simulink model "Disc_Integ_Forward_Euler_method_inherited_Sample_Time"  (R2014a)
settings: Solver=ode3  StartTime=0.0  StopTime=10.0  RelTol=1e-3
undefined symbols (not defined in the file): DiscIntNeverNeededParam
settings Model: CovSFcnEnable=on  Creator=bourbouh  LastModifiedBy=hbourbou
settings DataIOCC: LimitDataPoints=off  SaveFormat=StructureWithTime
settings DebuggingCC: MergeDetectMultiDrivingBlocksExec=error  SolverPrmCheckMsg=none  FrameProcessingCompatibilityMsg=error
settings HardwareCC: ProdBitPerPointer=64  ProdLargestAtomicFloat=Float  ProdIntDivRoundTo=Zero  ProdEndianess=LittleEndian  ProdHWDeviceType=Specified
settings ModelReferenceCC: PropagateSignalLabelsOutOfModel=on

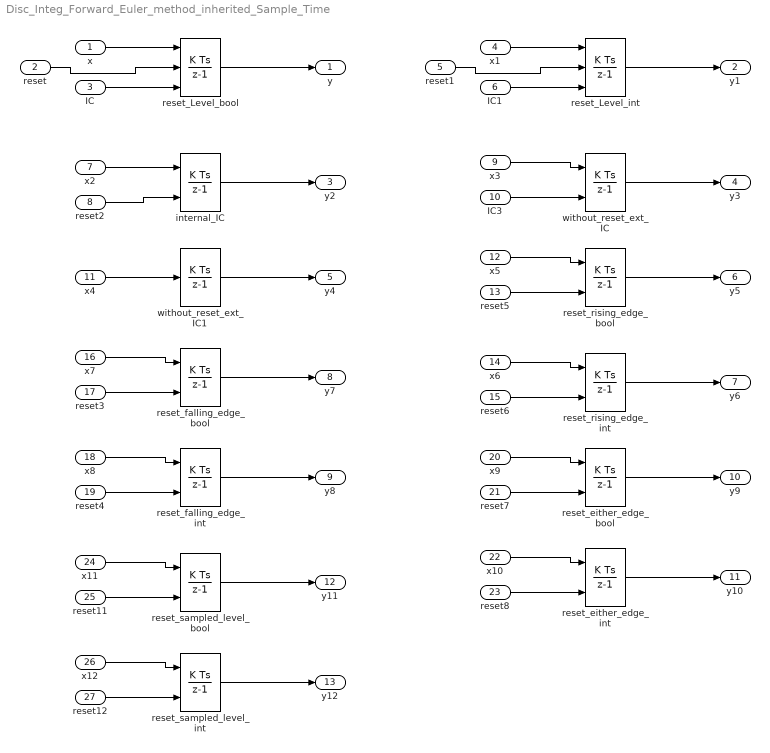
== system Disc_Integ_Forward_Euler_method_inherited_Sample_Time ==
  x : Inport
  reset : Inport  Port=2  OutDataTypeStr=boolean
  IC : Inport  Port=3
  x1 : Inport  Port=4
  reset1 : Inport  Port=5  OutDataTypeStr=int32
  IC1 : Inport  Port=6
  x2 : Inport  Port=7
  reset2 : Inport  Port=8  OutDataTypeStr=boolean
  x3 : Inport  Port=9
  IC3 : Inport  Port=10
  x4 : Inport  Port=11
  x5 : Inport  Port=12
  reset5 : Inport  Port=13  OutDataTypeStr=boolean
  x6 : Inport  Port=14
  reset6 : Inport  Port=15  OutDataTypeStr=int32
  x7 : Inport  Port=16
  reset3 : Inport  Port=17  OutDataTypeStr=boolean
  x8 : Inport  Port=18
  reset4 : Inport  Port=19  OutDataTypeStr=int32
  x9 : Inport  Port=20
  reset7 : Inport  Port=21  OutDataTypeStr=boolean
  x10 : Inport  Port=22
  reset8 : Inport  Port=23  OutDataTypeStr=int32
  x11 : Inport  Port=24
  reset11 : Inport  Port=25  OutDataTypeStr=boolean
  x12 : Inport  Port=26
  reset12 : Inport  Port=27  OutDataTypeStr=int32
  internal_IC : DiscreteIntegrator  ExternalReset=level  SampleTime=-1  ICPrevOutput=DiscIntNeverNeededParam  ICPrevScaledInput=DiscIntNeverNeededParam  mask(DiscretizedDiscreteIntegrator){}
      mask init:
      | %zoh
  reset_Level_bool : DiscreteIntegrator  ExternalReset=level  InitialConditionSource=external  SampleTime=-1  ICPrevOutput=DiscIntNeverNeededParam  ICPrevScaledInput=DiscIntNeverNeededParam  mask(DiscretizedDiscreteIntegrator){}
      mask init:
      | %zoh
  reset_Level_int : DiscreteIntegrator  ExternalReset=level  InitialConditionSource=external  SampleTime=-1  ICPrevOutput=DiscIntNeverNeededParam  ICPrevScaledInput=DiscIntNeverNeededParam  mask(DiscretizedDiscreteIntegrator){}
      mask init:
      | %zoh
  reset_either_edge_bool : DiscreteIntegrator  ExternalReset=either  SampleTime=-1  ICPrevOutput=DiscIntNeverNeededParam  ICPrevScaledInput=DiscIntNeverNeededParam  mask(DiscretizedDiscreteIntegrator){}
      mask init:
      | %zoh
  reset_either_edge_int : DiscreteIntegrator  ExternalReset=either  SampleTime=-1  ICPrevOutput=DiscIntNeverNeededParam  ICPrevScaledInput=DiscIntNeverNeededParam  mask(DiscretizedDiscreteIntegrator){}
      mask init:
      | %zoh
  reset_falling_edge_bool : DiscreteIntegrator  ExternalReset=falling  SampleTime=-1  ICPrevOutput=DiscIntNeverNeededParam  ICPrevScaledInput=DiscIntNeverNeededParam  mask(DiscretizedDiscreteIntegrator){}
      mask init:
      | %zoh
  reset_falling_edge_int : DiscreteIntegrator  ExternalReset=falling  SampleTime=-1  ICPrevOutput=DiscIntNeverNeededParam  ICPrevScaledInput=DiscIntNeverNeededParam  mask(DiscretizedDiscreteIntegrator){}
      mask init:
      | %zoh
  reset_rising_edge_bool : DiscreteIntegrator  ExternalReset=rising  SampleTime=-1  ICPrevOutput=DiscIntNeverNeededParam  ICPrevScaledInput=DiscIntNeverNeededParam  mask(DiscretizedDiscreteIntegrator){}
      mask init:
      | %zoh
  reset_rising_edge_int : DiscreteIntegrator  ExternalReset=rising  SampleTime=-1  ICPrevOutput=DiscIntNeverNeededParam  ICPrevScaledInput=DiscIntNeverNeededParam  mask(DiscretizedDiscreteIntegrator){}
      mask init:
      | %zoh
  reset_sampled_level_bool : DiscreteIntegrator  ExternalReset=sampled level  SampleTime=-1  ICPrevOutput=DiscIntNeverNeededParam  ICPrevScaledInput=DiscIntNeverNeededParam  mask(DiscretizedDiscreteIntegrator){}
      mask init:
      | %zoh
  reset_sampled_level_int : DiscreteIntegrator  ExternalReset=sampled level  SampleTime=-1  ICPrevOutput=DiscIntNeverNeededParam  ICPrevScaledInput=DiscIntNeverNeededParam  mask(DiscretizedDiscreteIntegrator){}
      mask init:
      | %zoh
  without_reset_ext_IC : DiscreteIntegrator  InitialConditionSource=external  SampleTime=-1  ICPrevOutput=DiscIntNeverNeededParam  ICPrevScaledInput=DiscIntNeverNeededParam  mask(DiscretizedDiscreteIntegrator){}
      mask init:
      | %zoh
  without_reset_ext_IC1 : DiscreteIntegrator  SampleTime=-1  ICPrevOutput=DiscIntNeverNeededParam  ICPrevScaledInput=DiscIntNeverNeededParam  mask(DiscretizedDiscreteIntegrator){}
      mask init:
      | %zoh
  y : Outport
  y1 : Outport  Port=2
  y2 : Outport  Port=3
  y3 : Outport  Port=4
  y4 : Outport  Port=5
  y5 : Outport  Port=6
  y6 : Outport  Port=7
  y7 : Outport  Port=8
  y8 : Outport  Port=9
  y9 : Outport  Port=10
  y10 : Outport  Port=11
  y11 : Outport  Port=12
  y12 : Outport  Port=13
  wires:
  x/1 -> reset_Level_bool/1
  IC/1 -> reset_Level_bool/3
  reset_Level_bool/1 -> y/1
  reset/1 -> reset_Level_bool/2
  x1/1 -> reset_Level_int/1
  IC1/1 -> reset_Level_int/3
  reset_Level_int/1 -> y1/1
  reset1/1 -> reset_Level_int/2
  x2/1 -> internal_IC/1
  internal_IC/1 -> y2/1
  reset2/1 -> internal_IC/2
  x3/1 -> without_reset_ext_IC/1
  IC3/1 -> without_reset_ext_IC/2
  without_reset_ext_IC/1 -> y3/1
  x4/1 -> without_reset_ext_IC1/1
  without_reset_ext_IC1/1 -> y4/1
  x5/1 -> reset_rising_edge_bool/1
  reset_rising_edge_bool/1 -> y5/1
  reset5/1 -> reset_rising_edge_bool/2
  x6/1 -> reset_rising_edge_int/1
  reset_rising_edge_int/1 -> y6/1
  reset6/1 -> reset_rising_edge_int/2
  x7/1 -> reset_falling_edge_bool/1
  reset_falling_edge_bool/1 -> y7/1
  reset3/1 -> reset_falling_edge_bool/2
  x8/1 -> reset_falling_edge_int/1
  reset_falling_edge_int/1 -> y8/1
  reset4/1 -> reset_falling_edge_int/2
  x9/1 -> reset_either_edge_bool/1
  reset_either_edge_bool/1 -> y9/1
  reset7/1 -> reset_either_edge_bool/2
  x10/1 -> reset_either_edge_int/1
  reset_either_edge_int/1 -> y10/1
  reset8/1 -> reset_either_edge_int/2
  x11/1 -> reset_sampled_level_bool/1
  reset_sampled_level_bool/1 -> y11/1
  reset11/1 -> reset_sampled_level_bool/2
  x12/1 -> reset_sampled_level_int/1
  reset_sampled_level_int/1 -> y12/1
  reset12/1 -> reset_sampled_level_int/2
